simulink model "eye_model"  (R2019a)
settings: Solver=FixedStepAuto  StartTime=t_start  StopTime=t_finish  FixedStep=fix_step_size/100  RelTol=1e-3
values from neighbouring files (symbols this model uses):
  B = 0.018    [EyeScript.m]
  fix_step_size = 0.001    [EyeScript.m]
  J = 4.3 * 10e-5    (= 0.00043)    [EyeScript.m]
  K = 0.86    [EyeScript.m]
  Kse = 1.8    [EyeScript.m]
  LeftAgInit = LeftAgStepPrev    [EyeScript.m]
  LeftAgPulse = LeftPh    [EyeScript.m]
  LeftAgPW = LeftPW    (= 0.04)    [EyeScript.m]
  LeftAgStep = LeftAgStepPrev+0.8*LeftDthetaValues(m)    [EyeScript.m]
  LeftAgStepPrev = LeftAgStepLog(m)    [EyeScript.m]
  LeftAntInit = LeftAntStepPrev    [EyeScript.m]
  LeftAntPulse = 0.5 + LeftAntStepPrev*exp(-LeftDthetaValues(m)/2.5)    [EyeScript.m]
  LeftAntPW = LeftAgPW; + 6e-3    [EyeScript.m]
  LeftAntStep = LeftAntStepPrev - 0.06*LeftDthetaValues(m)    [EyeScript.m]
  LeftAntStepPrev = LeftAntStepLog(m)    [EyeScript.m]
  LeftPW = 40e-3    (= 0.04)    [EyeScript.m]
  LeftTauAg_AC = (13 - 0.1*LeftDthetaValues(m))*1e-3    [EyeScript.m]
  LeftTheta1_init = LeftTheta1(end)    [EyeScript.m]
  LeftTheta1dot_init = LeftTheta1dot(end)    [EyeScript.m]
  LeftTheta2_init = LeftTheta2(end)    [EyeScript.m]
  LeftTheta3_init = LeftTheta3(end)    [EyeScript.m]
  RightAgInit = RightAgStepPrev    [EyeScript.m]
  RightAgPulse = RightPh    [EyeScript.m]
  RightAgPW = RightPW    (= 0.04)    [EyeScript.m]
  RightAgStep = RightAgStepPrev+0.8*RightDthetaValues(m)    [EyeScript.m]
  RightAgStepPrev = RightAgStepLog(m)    [EyeScript.m]
  RightAntInit = RightAntStepPrev    [EyeScript.m]
  RightAntPulse = 0.5 + RightAntStepPrev*exp(-RightDthetaValues(m)/2.5)    [EyeScript.m]
  RightAntPW = RightAgPW + 6e-3    (= 0.046)    [EyeScript.m]
  RightAntStep = RightAntStepPrev - 0.06*RightDthetaValues(m)    [EyeScript.m]
  RightAntStepPrev = RightAntStepLog(m)    [EyeScript.m]
  RightTauAg_AC = (13 - 0.1*RightDthetaValues(m))*1e-3    [EyeScript.m]
  RightTheta1_init = RightTheta1(end)    [EyeScript.m]
  RightTheta1dot_init = RightTheta1dot(end)    [EyeScript.m]
  RightTheta2_init = RightTheta2(end)    [EyeScript.m]
  RightTheta3_init = RightTheta3(end)    [EyeScript.m]
  zero = 5e-3    (= 0.005)    [EyeScript.m]
undefined symbols (not defined in the file or in its folder): PW, TauAG_AC
settings Model: Creator=murat  LastModifiedBy=murat

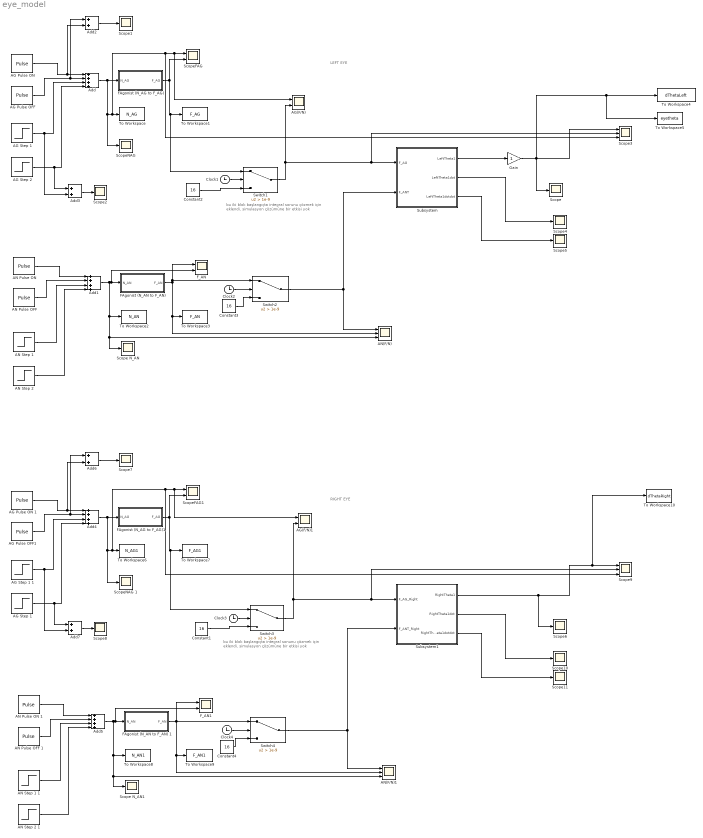
== system eye_model ==
  note: bu iki blok başlangıçta integral sonunu çözmek için eklendi, simulasyon çözümüne bir etkisi yok
  note: LEFT
      | EYE
  note: RIGHT
      | EYE
  note: bu iki blok başlangıçta integral sorunu çözmek için eklendi, simulasyon çözümüne bir etkisi yok
  AG Pulse OFF : DiscretePulseGenerator  PulseType=Time based  Amplitude=-LeftAgPulse  Period=2*LeftAgPW  PulseWidth=50  PhaseDelay=2*LeftPW+zero  VectorParams1D=off
  AG Pulse OFF1 : DiscretePulseGenerator  PulseType=Time based  Amplitude=-RightAgPulse  Period=2*RightAgPW  PulseWidth=50  PhaseDelay=2*RightAgPW+zero  VectorParams1D=off
  "AG Pulse ON " : DiscretePulseGenerator  PulseType=Time based  Amplitude=LeftAgPulse  Period=2*LeftAgPW  PulseWidth=50  PhaseDelay=zero  VectorParams1D=off
  AG Pulse ON 1 : DiscretePulseGenerator  PulseType=Time based  Amplitude=RightAgPulse  Period=2*RightAgPW  PulseWidth=50  PhaseDelay=zero  VectorParams1D=off
  AG Step 1 : Step  Time=zero + RightAgPW  After=RightAgStep  SampleTime=fix_step_size  VectorParams1D=off
  "AG Step 1 " : Step  Time=zero  Before=LeftAgStepPrev  After=0  SampleTime=fix_step_size  VectorParams1D=off  ZeroCross=off
  AG Step 1 1 : Step  Time=zero  Before=RightAgStepPrev  After=0  SampleTime=fix_step_size  VectorParams1D=off  ZeroCross=off
  AG Step 2 : Step  Time=zero + LeftPW  After=LeftAgStep  SampleTime=fix_step_size  VectorParams1D=off
  AG(F/N) : Scope  NumInputPorts=2
  AG(F/N)1 : Scope  NumInputPorts=2
  "AN Pulse OFF " : DiscretePulseGenerator  PulseType=Time based  Amplitude=-LeftAntPulse  Period=2*LeftAntPW  PulseWidth=50  PhaseDelay=2*LeftAntPW+zero-(3e-3)  VectorParams1D=off
  AN Pulse OFF 1 : DiscretePulseGenerator  PulseType=Time based  Amplitude=-RightAntPulse  Period=2*RightAntPW  PulseWidth=50  PhaseDelay=2*RightAntPW+zero-(3e-3)  VectorParams1D=off
  "AN Pulse ON " : DiscretePulseGenerator  PulseType=Time based  Amplitude=LeftAntPulse  Period=2*LeftAntPW  PulseWidth=50  PhaseDelay=zero-(3e-3)  VectorParams1D=off
  AN Pulse ON 1 : DiscretePulseGenerator  PulseType=Time based  Amplitude=RightAntPulse  Period=2*RightAntPW  PulseWidth=50  PhaseDelay=zero-(3e-3)  VectorParams1D=off
  "AN Step 1 " : Step  Time=zero-3e-3  Before=LeftAntStepPrev  After=0  SampleTime=fix_step_size
  AN Step 1 1 : Step  Time=zero-3e-3  Before=RightAntStepPrev  After=0  SampleTime=fix_step_size
  "AN Step 2 " : Step  Time=zero + LeftAntPW - 3e-3  After=LeftAntStep  SampleTime=fix_step_size
  AN Step 2 1 : Step  Time=zero + RightAntPW - 3e-3  After=RightAntStep  SampleTime=fix_step_size
  AN(F/N) : Scope  NumInputPorts=3
  AN(F/N)1 : Scope  NumInputPorts=3
  Add{,1,4..5} (4 alike) : Sum  Inputs=++++
  Add{2..3,6..7} (4 alike) : Sum
  Clock{1..4} (4 alike) : Clock
  Constant{1..4} (4 alike) : Constant  Value=16
  FAgonist (N_AG to F_AG) : Subsystem
  FAgonist (N_AG to F_AG)1 : Subsystem
  "FAgonist (N_AN to F_AN) " : Subsystem
  FAgonist (N_AN to F_AN) 1 : Subsystem
  F_AN : Scope  NumInputPorts=2
  F_AN1 : Scope  NumInputPorts=2
  Gain : Gain
  Scope{,1..2,4..8,10..11} (10 alike) : Scope
  Scope N_AN : Scope
  Scope N_AN1 : Scope
  Scope3 : Scope  NumInputPorts=3
  Scope9 : Scope  NumInputPorts=3
  ScopeFAG : Scope  NumInputPorts=2
  ScopeFAG1 : Scope  NumInputPorts=2
  "ScopeNAG " : Scope
  ScopeNAG 1 : Scope
  Subsystem : Subsystem
  Subsystem1 : Subsystem
  Switch{1..4} (4 alike) : Switch  Criteria=u2 > Threshold  Threshold=1e-9
  To Workspace : ToWorkspace  VariableName=N_AG  SaveFormat=Timeseries  SampleTime=-1
  To Workspace1 : ToWorkspace  VariableName=F_AG  SaveFormat=Timeseries  SampleTime=-1
  To Workspace10 : ToWorkspace  VariableName=dThetaRight  SampleTime=-1
  To Workspace2 : ToWorkspace  VariableName=N_AN  SaveFormat=Timeseries  SampleTime=-1
  To Workspace3 : ToWorkspace  VariableName=F_AN  SaveFormat=Timeseries  SampleTime=-1
  To Workspace4 : ToWorkspace  VariableName=dThetaLeft  SampleTime=-1
  To Workspace5 : ToWorkspace  VariableName=eyetheta  SaveFormat=Timeseries  SampleTime=-1
  To Workspace6 : ToWorkspace  VariableName=N_AG1  SaveFormat=Timeseries  SampleTime=-1
  To Workspace7 : ToWorkspace  VariableName=F_AG1  SaveFormat=Timeseries  SampleTime=-1
  To Workspace8 : ToWorkspace  VariableName=N_AN1  SaveFormat=Timeseries  SampleTime=-1
  To Workspace9 : ToWorkspace  VariableName=F_AN1  SaveFormat=Timeseries  SampleTime=-1
  wires:
  "AG Pulse ON "/1 -> Add2/2, Add/1
  Add/1 -> Scope3/3, AG(F/N)/1, ScopeFAG/1, To Workspace/1, "ScopeNAG "/1, FAgonist (N_AG to F_AG)/1(N_AG)
  "AG Step 1 "/1 -> Add3/2, Add/3
  AG Pulse OFF/1 -> Add2/1, Add/2
  FAgonist (N_AG to F_AG)/1(F_AG) -> Switch1/1, To Workspace1/1, ScopeFAG/2
  "FAgonist (N_AN to F_AN) "/1(F_AN) -> F_AN/1, Switch2/1, AN(F/N)/2, To Workspace3/1
  "AN Pulse OFF "/1 -> Add1/2
  Add1/1 -> To Workspace2/1, Scope N_AN/1, AN(F/N)/3, F_AN/2, "FAgonist (N_AN to F_AN) "/1(N_AN)
  "AN Pulse ON "/1 -> Add1/1
  AG Step 2/1 -> Add3/1, Add/4
  "AN Step 1 "/1 -> Add1/3
  "AN Step 2 "/1 -> Add1/4
  Clock1/1 -> Switch1/2
  Switch1/1 -> AG(F/N)/2, Scope3/2, Subsystem/1(F_AG)
  Constant2/1 -> Switch1/3
  Clock2/1 -> Switch2/2
  Constant3/1 -> Switch2/3
  Switch2/1 -> AN(F/N)/1, Subsystem/2(F_ANT)
  Subsystem/2(LeftTheta1dot) -> Scope4/1
  Subsystem/3(LeftTheta1dotdot) -> Scope5/1
  Subsystem/1(LeftTheta1) -> Gain/1
  Gain/1 -> Scope/1, To Workspace5/1, To Workspace4/1, Scope3/1
  Add2/1 -> Scope1/1
  Add3/1 -> Scope2/1
  Add7/1 -> Scope8/1
  Add6/1 -> Scope7/1
  Subsystem1/1(RightTheta1) -> To Workspace10/1, Scope9/1, Scope6/1
  Subsystem1/3(RightTheta1dotdot) -> Scope11/1
  Subsystem1/2(RightTheta1dot) -> Scope10/1
  Switch4/1 -> Subsystem1/2("F_ANT_Right "), AN(F/N)1/1
  Constant4/1 -> Switch4/3
  Clock4/1 -> Switch4/2
  Constant1/1 -> Switch3/3
  Switch3/1 -> AG(F/N)1/2, Subsystem1/1(F_AG_Right), Scope9/2
  Clock3/1 -> Switch3/2
  AN Step 2 1/1 -> Add5/4
  AN Step 1 1/1 -> Add5/3
  AG Step 1/1 -> Add4/4, Add7/1
  AN Pulse ON 1/1 -> Add5/1
  Add5/1 -> FAgonist (N_AN to F_AN) 1/1(N_AN), F_AN1/2, AN(F/N)1/3, Scope N_AN1/1, To Workspace8/1
  AN Pulse OFF 1/1 -> Add5/2
  FAgonist (N_AN to F_AN) 1/1(F_AN) -> To Workspace9/1, AN(F/N)1/2, Switch4/1, F_AN1/1
  FAgonist (N_AG to F_AG)1/1(F_AG) -> ScopeFAG1/2, To Workspace7/1, Switch3/1
  AG Pulse OFF1/1 -> Add4/2, Add6/1
  AG Step 1 1/1 -> Add4/3, Add7/2
  Add4/1 -> FAgonist (N_AG to F_AG)1/1(N_AG), ScopeNAG 1/1, To Workspace6/1, ScopeFAG1/1, AG(F/N)1/1, Scope9/3
  AG Pulse ON 1/1 -> Add4/1, Add6/2

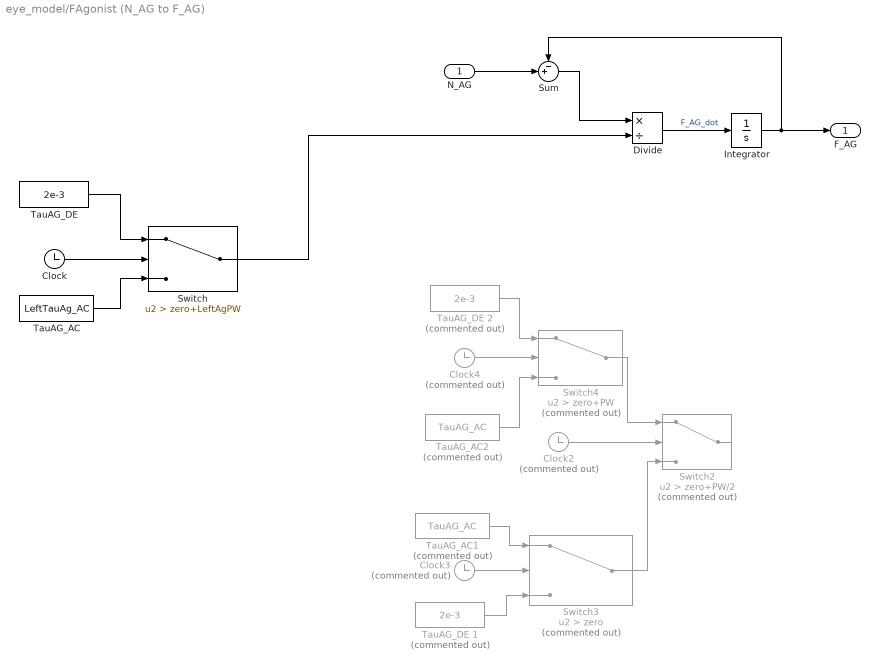
== system eye_model/FAgonist (N_AG to F_AG) ==
  N_AG : Inport
  Clock : Clock
  Clock2 : Clock  Commented=on
  Clock3 : Clock  Commented=on
  Clock4 : Clock  Commented=on
  Divide : Product  Inputs=*/
  Integrator : Integrator  InitialCondition=LeftAgInit
  Sum : Sum  Inputs=-+|
  Switch : Switch  Criteria=u2 > Threshold  Threshold=zero+LeftAgPW
  Switch2 : Switch  Commented=on  Criteria=u2 > Threshold  Threshold=zero+PW/2
  Switch3 : Switch  Commented=on  Criteria=u2 > Threshold  Threshold=zero
  Switch4 : Switch  Commented=on  Criteria=u2 > Threshold  Threshold=zero+PW
  TauAG_AC : Constant  Value=LeftTauAg_AC
  TauAG_AC1 : Constant  Commented=on  Value=TauAG_AC
  TauAG_AC2 : Constant  Commented=on  Value=TauAG_AC
  "TauAG_DE " : Constant  Value=2e-3
  TauAG_DE 1 : Constant  Commented=on  Value=2e-3
  TauAG_DE 2 : Constant  Commented=on  Value=2e-3
  F_AG : Outport
  wires:
  Clock/1 -> Switch/2
  N_AG/1 -> Sum/2
  Sum/1 -> Divide/1
  Divide/1 -> Integrator/1  "F_AG_dot"
  Integrator/1 -> Sum/1, F_AG/1
  Clock2/1 -> Switch2/2
  TauAG_AC/1 -> Switch/3
  "TauAG_DE "/1 -> Switch/1
  Switch4/1 -> Switch2/1
  Switch3/1 -> Switch2/3
  TauAG_DE 2/1 -> Switch4/1
  TauAG_AC2/1 -> Switch4/3
  Clock4/1 -> Switch4/2
  Clock3/1 -> Switch3/2
  TauAG_DE 1/1 -> Switch3/3
  TauAG_AC1/1 -> Switch3/1
  Switch/1 -> Divide/2

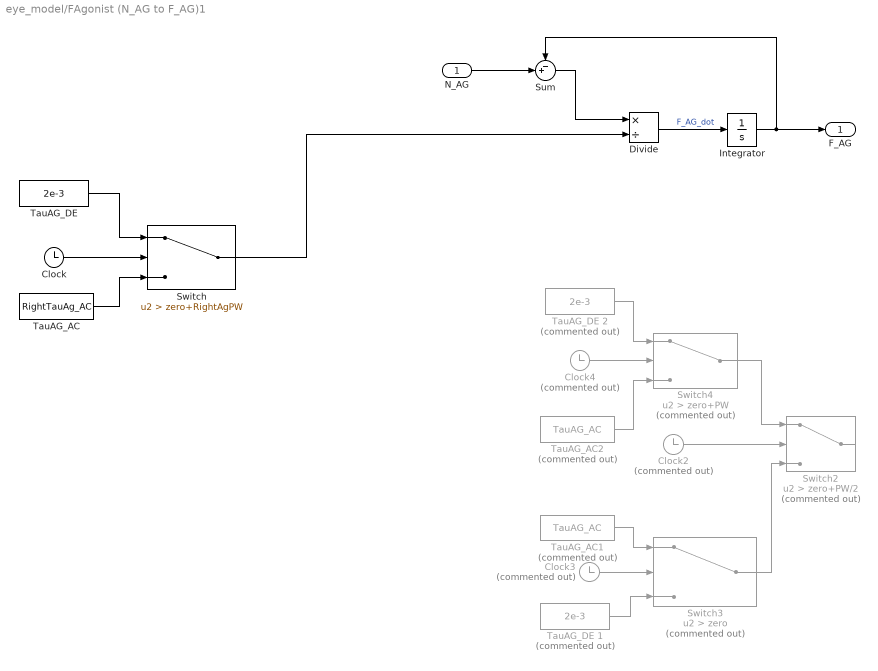
== system eye_model/FAgonist (N_AG to F_AG)1 ==
  N_AG : Inport
  Clock : Clock
  Clock2 : Clock  Commented=on
  Clock3 : Clock  Commented=on
  Clock4 : Clock  Commented=on
  Divide : Product  Inputs=*/
  Integrator : Integrator  InitialCondition=RightAgInit
  Sum : Sum  Inputs=-+|
  Switch : Switch  Criteria=u2 > Threshold  Threshold=zero+RightAgPW
  Switch2 : Switch  Commented=on  Criteria=u2 > Threshold  Threshold=zero+PW/2
  Switch3 : Switch  Commented=on  Criteria=u2 > Threshold  Threshold=zero
  Switch4 : Switch  Commented=on  Criteria=u2 > Threshold  Threshold=zero+PW
  TauAG_AC : Constant  Value=RightTauAg_AC
  TauAG_AC1 : Constant  Commented=on  Value=TauAG_AC
  TauAG_AC2 : Constant  Commented=on  Value=TauAG_AC
  "TauAG_DE " : Constant  Value=2e-3
  TauAG_DE 1 : Constant  Commented=on  Value=2e-3
  TauAG_DE 2 : Constant  Commented=on  Value=2e-3
  F_AG : Outport
  wires:
  Switch/1 -> Divide/2
  TauAG_AC1/1 -> Switch3/1
  TauAG_DE 1/1 -> Switch3/3
  Clock3/1 -> Switch3/2
  Clock4/1 -> Switch4/2
  TauAG_AC2/1 -> Switch4/3
  TauAG_DE 2/1 -> Switch4/1
  Switch3/1 -> Switch2/3
  Switch4/1 -> Switch2/1
  "TauAG_DE "/1 -> Switch/1
  TauAG_AC/1 -> Switch/3
  Clock2/1 -> Switch2/2
  Integrator/1 -> F_AG/1, Sum/1
  Divide/1 -> Integrator/1  "F_AG_dot"
  Sum/1 -> Divide/1
  N_AG/1 -> Sum/2
  Clock/1 -> Switch/2

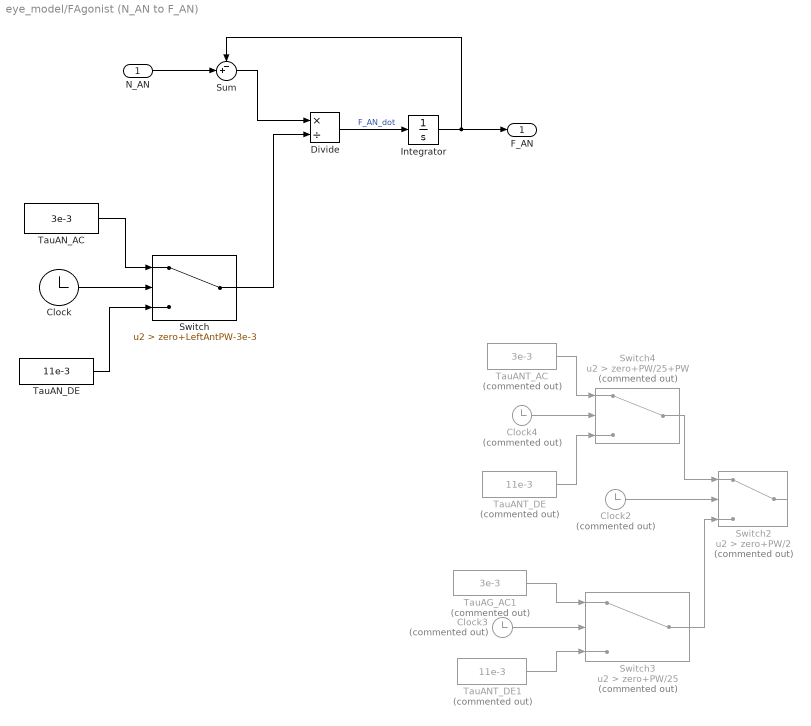
== system eye_model/FAgonist (N_AN to F_AN)  ==
  N_AN : Inport
  Clock : Clock
  Clock2 : Clock  Commented=on
  Clock3 : Clock  Commented=on
  Clock4 : Clock  Commented=on
  Divide : Product  Inputs=*/
  Integrator : Integrator  InitialCondition=LeftAntInit
  Sum : Sum  Inputs=-+|
  Switch : Switch  Criteria=u2 > Threshold  Threshold=zero+LeftAntPW-3e-3
  Switch2 : Switch  Commented=on  Criteria=u2 > Threshold  Threshold=zero+PW/2
  Switch3 : Switch  Commented=on  Criteria=u2 > Threshold  Threshold=zero+PW/25
  Switch4 : Switch  Commented=on  Criteria=u2 > Threshold  Threshold=zero+PW/25+PW
  TauAG_AC1 : Constant  Commented=on  Value=3e-3
  TauANT_AC : Constant  Commented=on  Value=3e-3
  TauANT_DE : Constant  Commented=on  Value=11e-3
  TauANT_DE1 : Constant  Commented=on  Value=11e-3
  "TauAN_AC " : Constant  Value=3e-3
  TauAN_DE : Constant  Value=11e-3
  F_AN : Outport
  wires:
  Clock/1 -> Switch/2
  "TauAN_AC "/1 -> Switch/1
  TauAN_DE/1 -> Switch/3
  Sum/1 -> Divide/1
  Divide/1 -> Integrator/1  "F_AN_dot"
  Integrator/1 -> Sum/1, F_AN/1
  N_AN/1 -> Sum/2
  Clock2/1 -> Switch2/2
  TauANT_DE1/1 -> Switch3/3
  TauAG_AC1/1 -> Switch3/1
  Switch3/1 -> Switch2/3
  Switch4/1 -> Switch2/1
  Clock3/1 -> Switch3/2
  Clock4/1 -> Switch4/2
  TauANT_DE/1 -> Switch4/3
  TauANT_AC/1 -> Switch4/1
  Switch/1 -> Divide/2

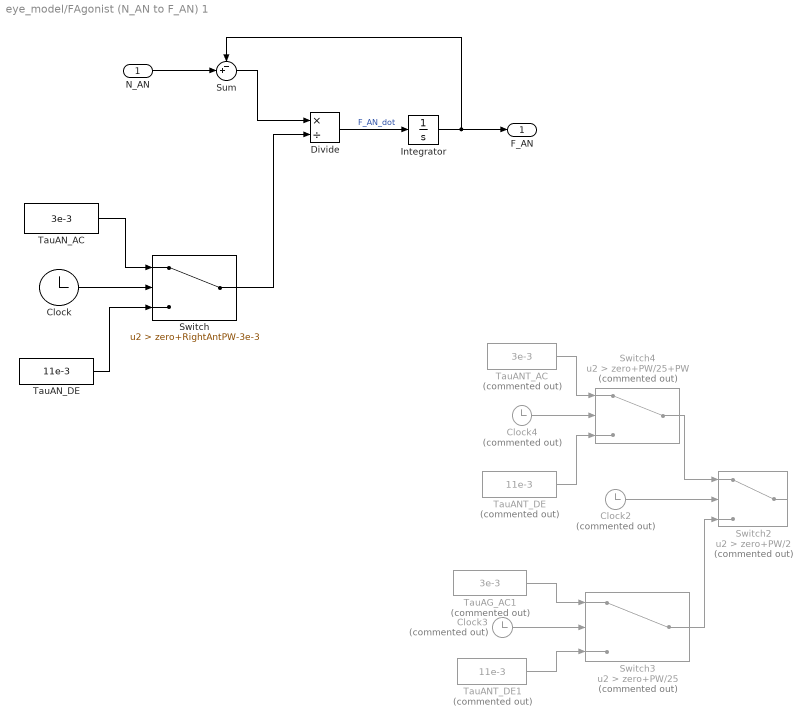
== system eye_model/FAgonist (N_AN to F_AN) 1 ==
  N_AN : Inport
  Clock : Clock
  Clock2 : Clock  Commented=on
  Clock3 : Clock  Commented=on
  Clock4 : Clock  Commented=on
  Divide : Product  Inputs=*/
  Integrator : Integrator  InitialCondition=RightAntInit
  Sum : Sum  Inputs=-+|
  Switch : Switch  Criteria=u2 > Threshold  Threshold=zero+RightAntPW-3e-3
  Switch2 : Switch  Commented=on  Criteria=u2 > Threshold  Threshold=zero+PW/2
  Switch3 : Switch  Commented=on  Criteria=u2 > Threshold  Threshold=zero+PW/25
  Switch4 : Switch  Commented=on  Criteria=u2 > Threshold  Threshold=zero+PW/25+PW
  TauAG_AC1 : Constant  Commented=on  Value=3e-3
  TauANT_AC : Constant  Commented=on  Value=3e-3
  TauANT_DE : Constant  Commented=on  Value=11e-3
  TauANT_DE1 : Constant  Commented=on  Value=11e-3
  "TauAN_AC " : Constant  Value=3e-3
  TauAN_DE : Constant  Value=11e-3
  F_AN : Outport
  wires:
  Switch/1 -> Divide/2
  TauANT_AC/1 -> Switch4/1
  TauANT_DE/1 -> Switch4/3
  Clock4/1 -> Switch4/2
  Clock3/1 -> Switch3/2
  Switch4/1 -> Switch2/1
  Switch3/1 -> Switch2/3
  TauAG_AC1/1 -> Switch3/1
  TauANT_DE1/1 -> Switch3/3
  Clock2/1 -> Switch2/2
  N_AN/1 -> Sum/2
  Integrator/1 -> F_AN/1, Sum/1
  Divide/1 -> Integrator/1  "F_AN_dot"
  Sum/1 -> Divide/1
  TauAN_DE/1 -> Switch/3
  "TauAN_AC "/1 -> Switch/1
  Clock/1 -> Switch/2

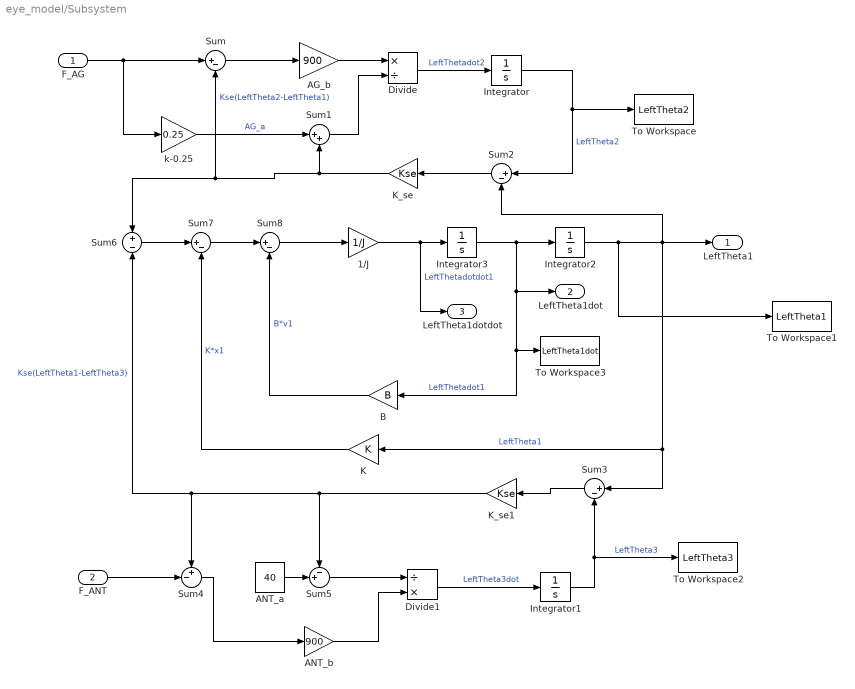
== system eye_model/Subsystem ==
  F_AG : Inport
  F_ANT : Inport  Port=2
  1/J : Gain  Gain=1/J
  AG_b : Gain  Gain=900
  ANT_a : Constant  Value=40
  ANT_b : Gain  Gain=900
  B : Gain  Gain=B
  Divide : Product  Inputs=*/
  Divide1 : Product  Inputs=/*
  Integrator : Integrator  InitialCondition=LeftTheta2_init
  Integrator1 : Integrator  InitialCondition=LeftTheta3_init
  Integrator2 : Integrator  InitialCondition=LeftTheta1_init
  Integrator3 : Integrator  InitialCondition=LeftTheta1dot_init
  "K " : Gain  Gain=K
  K_se : Gain  Gain=Kse
  "K_se1 " : Gain  Gain=Kse
  Sum{,2..3,7..8} (5 alike) : Sum  Inputs=|+-
  Sum1 : Sum  Inputs=|++
  Sum4 : Sum  Inputs=+-|
  Sum5 : Sum  Inputs=-+|
  Sum6 : Sum  Inputs=+|-
  To Workspace : ToWorkspace  VariableName=LeftTheta2  SaveFormat=Timeseries  SampleTime=-1
  To Workspace1 : ToWorkspace  VariableName=LeftTheta1  SaveFormat=Timeseries  SampleTime=-1
  To Workspace2 : ToWorkspace  VariableName=LeftTheta3  SaveFormat=Timeseries  SampleTime=-1
  To Workspace3 : ToWorkspace  VariableName=LeftTheta1dot  SaveFormat=Timeseries  SampleTime=-1
  k-0.25 : Gain  Gain=0.25
  LeftTheta1 : Outport
  LeftTheta1dot : Outport  Port=2
  LeftTheta1dotdot : Outport  Port=3
  wires:
  F_AG/1 -> k-0.25/1, Sum/1
  Sum/1 -> AG_b/1
  AG_b/1 -> Divide/1
  k-0.25/1 -> Sum1/1  "AG_a"
  Sum1/1 -> Divide/2
  Divide/1 -> Integrator/1  "LeftThetadot2"
  Integrator/1 -> To Workspace/1, Sum2/1  "LeftTheta2"
  Integrator2/1 -> To Workspace1/1, Sum2/2, Sum3/1, "K "/1, LeftTheta1/1  "LeftTheta1"
  Sum2/1 -> K_se/1
  K_se/1 -> Sum6/1, Sum/2, Sum1/2  "Kse(LeftTheta2-LeftTheta1)"
  Integrator1/1 -> To Workspace2/1, Sum3/2  "LeftTheta3"
  Divide1/1 -> Integrator1/1  "LeftTheta3dot"
  Sum3/1 -> "K_se1 "/1
  "K_se1 "/1 -> Sum5/1, Sum4/1, Sum6/2  "Kse(LeftTheta1-LeftTheta3)"
  F_ANT/1 -> Sum4/2
  ANT_a/1 -> Sum5/2
  Sum4/1 -> ANT_b/1
  Sum5/1 -> Divide1/1
  ANT_b/1 -> Divide1/2
  Integrator3/1 -> To Workspace3/1, B/1, LeftTheta1dot/1, Integrator2/1  "LeftThetadot1"
  1/J/1 -> LeftTheta1dotdot/1, Integrator3/1  "LeftThetadotdot1"
  Sum6/1 -> Sum7/1
  "K "/1 -> Sum7/2  "K*x1"
  B/1 -> Sum8/2  "B*v1"
  Sum7/1 -> Sum8/1
  Sum8/1 -> 1/J/1

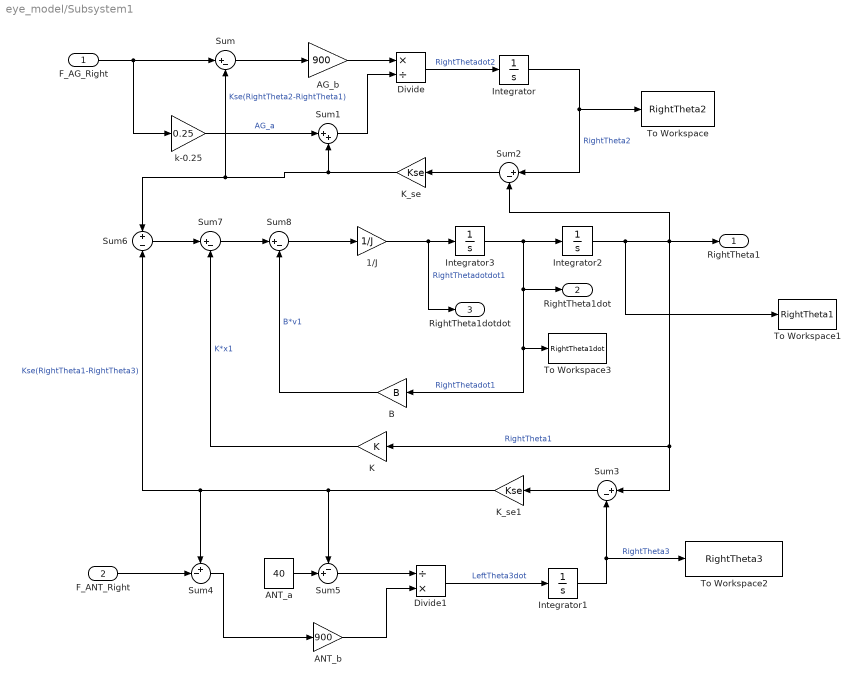
== system eye_model/Subsystem1 ==
  F_AG_Right : Inport
  "F_ANT_Right " : Inport  Port=2
  1/J : Gain  Gain=1/J
  AG_b : Gain  Gain=900
  ANT_a : Constant  Value=40
  ANT_b : Gain  Gain=900
  B : Gain  Gain=B
  Divide : Product  Inputs=*/
  Divide1 : Product  Inputs=/*
  Integrator : Integrator  InitialCondition=RightTheta2_init
  Integrator1 : Integrator  InitialCondition=RightTheta3_init
  Integrator2 : Integrator  InitialCondition=RightTheta1_init
  Integrator3 : Integrator  InitialCondition=RightTheta1dot_init
  "K " : Gain  Gain=K
  K_se : Gain  Gain=Kse
  "K_se1 " : Gain  Gain=Kse
  Sum{,2..3,7..8} (5 alike) : Sum  Inputs=|+-
  Sum1 : Sum  Inputs=|++
  Sum4 : Sum  Inputs=+-|
  Sum5 : Sum  Inputs=-+|
  Sum6 : Sum  Inputs=+|-
  To Workspace : ToWorkspace  VariableName=RightTheta2  SaveFormat=Timeseries  SampleTime=-1
  To Workspace1 : ToWorkspace  VariableName=RightTheta1  SaveFormat=Timeseries  SampleTime=-1
  To Workspace2 : ToWorkspace  VariableName=RightTheta3  SaveFormat=Timeseries  SampleTime=-1
  To Workspace3 : ToWorkspace  VariableName=RightTheta1dot  SaveFormat=Timeseries  SampleTime=-1
  k-0.25 : Gain  Gain=0.25
  RightTheta1 : Outport
  RightTheta1dot : Outport  Port=2
  RightTheta1dotdot : Outport  Port=3
  wires:
  Sum8/1 -> 1/J/1
  Sum7/1 -> Sum8/1
  B/1 -> Sum8/2  "B*v1"
  "K "/1 -> Sum7/2  "K*x1"
  Sum6/1 -> Sum7/1
  1/J/1 -> Integrator3/1, RightTheta1dotdot/1  "RightThetadotdot1"
  Integrator3/1 -> Integrator2/1, RightTheta1dot/1, B/1, To Workspace3/1  "RightThetadot1"
  ANT_b/1 -> Divide1/2
  Sum5/1 -> Divide1/1
  Sum4/1 -> ANT_b/1
  ANT_a/1 -> Sum5/2
  "F_ANT_Right "/1 -> Sum4/2
  "K_se1 "/1 -> Sum6/2, Sum4/1, Sum5/1  "Kse(RightTheta1-RightTheta3)"
  Sum3/1 -> "K_se1 "/1
  Divide1/1 -> Integrator1/1  "LeftTheta3dot"
  Integrator1/1 -> Sum3/2, To Workspace2/1  "RightTheta3"
  K_se/1 -> Sum1/2, Sum/2, Sum6/1  "Kse(RightTheta2-RightTheta1)"
  Sum2/1 -> K_se/1
  Integrator2/1 -> RightTheta1/1, "K "/1, Sum3/1, Sum2/2, To Workspace1/1  "RightTheta1"
  Integrator/1 -> Sum2/1, To Workspace/1  "RightTheta2"
  Divide/1 -> Integrator/1  "RightThetadot2"
  Sum1/1 -> Divide/2
  k-0.25/1 -> Sum1/1  "AG_a"
  AG_b/1 -> Divide/1
  Sum/1 -> AG_b/1
  F_AG_Right/1 -> Sum/1, k-0.25/1
